simulink model "CLE1"  (R2019b)
settings: Solver=VariableStepAuto  StartTime=0.0  StopTime=50.0  MaxStep=.025  RelTol=1e-3
settings Model: OrderedModelArguments=off  Creator=Tris  LastModifiedBy=Tris

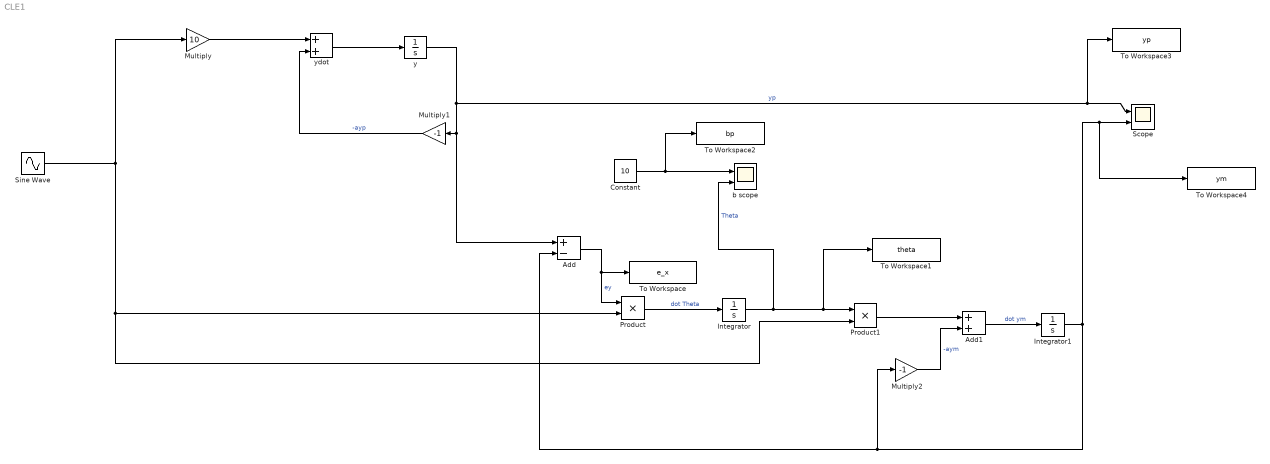
== system CLE1 ==
  Add : Sum  Inputs=+-
  Add1 : Sum
  Constant : Constant  Value=10
  Integrator : Integrator
  Integrator1 : Integrator
  Multiply : Gain  Gain=10
  Multiply1 : Gain  Gain=-1
  Multiply2 : Gain  Gain=-1
  Product : Product
  Product1 : Product
  Scope : Scope  NumInputPorts=2
  Sine Wave : Sin  SampleTime=0
  To Workspace : ToWorkspace  VariableName=e_x  SaveFormat=Timeseries  SampleTime=-1
  To Workspace1 : ToWorkspace  VariableName=theta  SaveFormat=Timeseries  SampleTime=-1
  To Workspace2 : ToWorkspace  VariableName=bp  SaveFormat=Timeseries  SampleTime=-1
  To Workspace3 : ToWorkspace  VariableName=yp  SaveFormat=Timeseries  SampleTime=-1
  To Workspace4 : ToWorkspace  VariableName=ym  SaveFormat=Timeseries  SampleTime=-1
  b scope : Scope  NumInputPorts=2
  y : Integrator
  ydot : Sum
  wires:
  Multiply/1 -> ydot/1
  ydot/1 -> y/1
  y/1 -> Add/1, Multiply1/1, To Workspace3/1, Scope/1  "yp"
  Multiply1/1 -> ydot/2  "-ayp"
  Add/1 -> Product/1, To Workspace/1  "ey"
  Product/1 -> Integrator/1  "dot Theta"
  Integrator/1 -> b scope/2, To Workspace1/1, Product1/1  "Theta"
  Product1/1 -> Add1/1
  Multiply2/1 -> Add1/2  "-aym"
  Add1/1 -> Integrator1/1  "dot ym"
  Integrator1/1 -> Add/2, Multiply2/1, To Workspace4/1, Scope/2
  Constant/1 -> To Workspace2/1, b scope/1
  Sine Wave/1 -> Multiply/1, Product1/2, Product/2
